simulink model "zy7gyz22"  (R2022a)
settings: Solver=VariableStepAuto  StartTime=0.0  StopTime=2.5  RelTol=1e-3
settings Model: Creator=dell  LastModifiedBy=dell

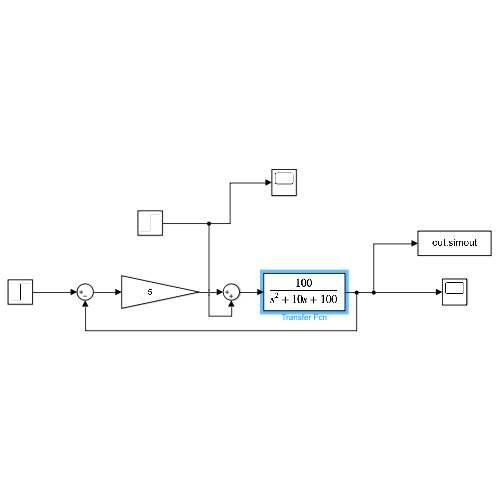
[thumbnail: Simulink's stored preview of the top-level diagram]
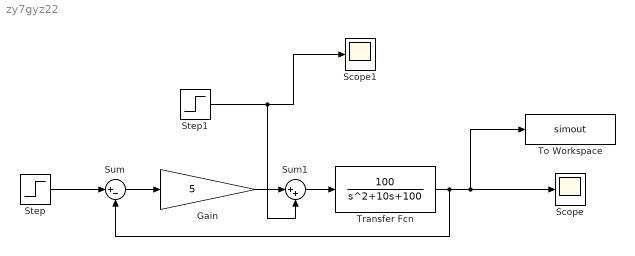
== system zy7gyz22 ==
  Gain : Gain  Gain=5
  Scope : Scope
  Scope1 : Scope
  Step : Step  Time=0  SampleTime=0
  Step1 : Step  SampleTime=0
  Sum : Sum  Inputs=|+-
  Sum1 : Sum  Inputs=|++
  To Workspace : ToWorkspace  VariableName=simout  SaveFormat=Timeseries  SampleTime=-1
  Transfer Fcn : TransferFcn  Numerator=[100]  Denominator=[1, 10, 100]
  wires:
  Step/1 -> Sum/1
  Transfer Fcn/1 -> Scope/1, To Workspace/1, Sum/2
  Sum/1 -> Gain/1
  Sum1/1 -> Transfer Fcn/1
  Gain/1 -> Sum1/1
  Step1/1 -> Sum1/2, Scope1/1
